simulink model "discret_line_systemm"  (R2022a)
settings: Solver=VariableStepAuto  StartTime=0.0  StopTime=1  RelTol=1e-8
values from neighbouring files (symbols this model uses):
  D = expm(A*T)    [discret_line_system.m]
undefined symbols (not defined in the file or in its folder): Xmax
settings Model: Creator=anyus  LastModifiedBy=anyus

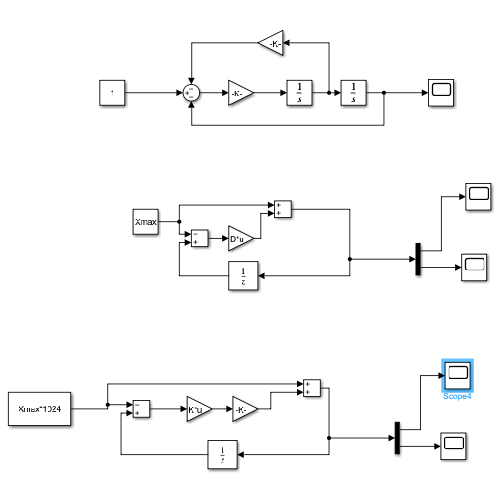
[thumbnail: Simulink's stored preview of the top-level diagram]
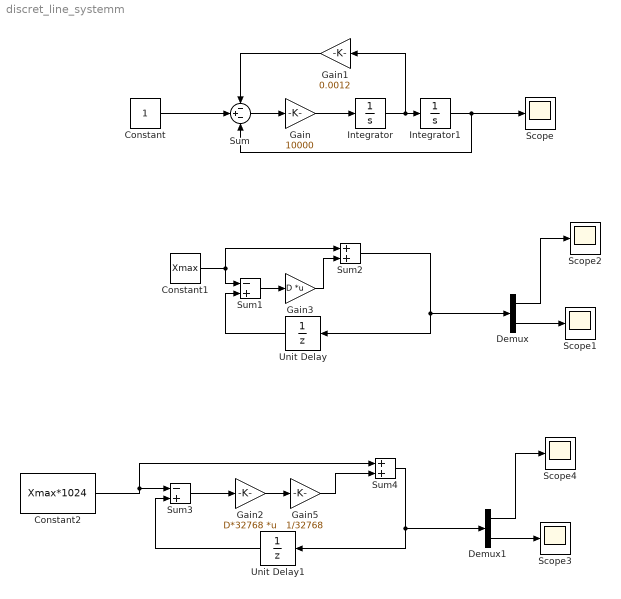
== system discret_line_systemm ==
  Constant : Constant
  Constant1 : Constant  Value=Xmax
  Constant2 : Constant  Value=Xmax*1024
  Demux : Demux  Outputs=2
  Demux1 : Demux  Outputs=2
  Gain : Gain  Gain=10000
  Gain1 : Gain  Gain=0.0012
  Gain2 : Gain  Gain=D*32768  Multiplication=Matrix(K*u)
  Gain3 : Gain  Gain=D  Multiplication=Matrix(K*u)
  Gain5 : Gain  Gain=1/32768
  Integrator : Integrator
  Integrator1 : Integrator
  Scope{,1..4} (5 alike) : Scope
  Sum : Sum  Inputs=-+-
  Sum1 : Sum  Inputs=-+
  Sum2 : Sum
  Sum3 : Sum  Inputs=-+
  Sum4 : Sum
  Unit Delay : UnitDelay  SampleTime=0.001  HasFrameUpgradeWarning=on
  Unit Delay1 : UnitDelay  SampleTime=0.001  HasFrameUpgradeWarning=on
  wires:
  Sum/1 -> Gain/1
  Integrator/1 -> Gain1/1, Integrator1/1
  Integrator1/1 -> Sum/3, Scope/1
  Gain/1 -> Integrator/1
  Constant/1 -> Sum/2
  Gain1/1 -> Sum/1
  Constant1/1 -> Sum2/1, Sum1/1
  Sum2/1 -> Demux/1, Unit Delay/1
  Unit Delay/1 -> Sum1/2
  Sum1/1 -> Gain3/1
  Gain3/1 -> Sum2/2
  Demux/2 -> Scope1/1
  Demux/1 -> Scope2/1
  Demux1/1 -> Scope4/1
  Demux1/2 -> Scope3/1
  Unit Delay1/1 -> Sum3/2
  Gain2/1 -> Gain5/1
  Sum3/1 -> Gain2/1
  Sum4/1 -> Demux1/1, Unit Delay1/1
  Constant2/1 -> Sum4/1, Sum3/1
  Gain5/1 -> Sum4/2
